simulink model "W05_S1"  (R2024b)
settings: Solver=ode4  StartTime=0  StopTime=T_final  FixedStep=h  RelTol=1e-3
values from neighbouring files (symbols this model uses):
  Delta = 8    [W05_S_expected.m]
  x0 = zeros(12,1);  x0(8) = V.y0;  assignin(b,'x0',x0)    [W05_S_expected.m]
undefined symbols (not defined in the file or in its folder): beta_c, k_neg, k_pos, Kd, Kp, law, mp, n_max, n_min, rp, V_c, WP_E, WP_N, X_ff, y_pont
settings Model: Creator=admin  LastModifiedBy=admin
settings DataIOCC: ReturnWorkspaceOutputs=off

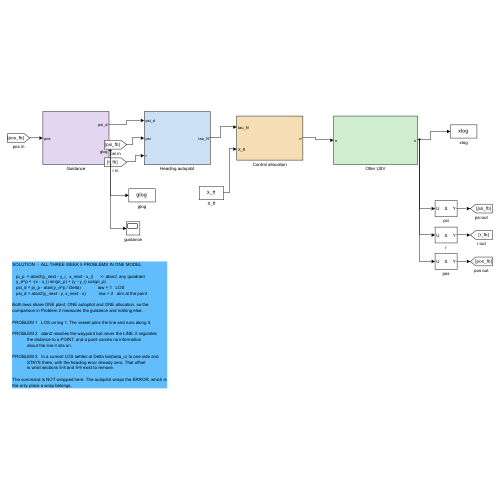
[thumbnail: Simulink's stored preview of the top-level diagram]
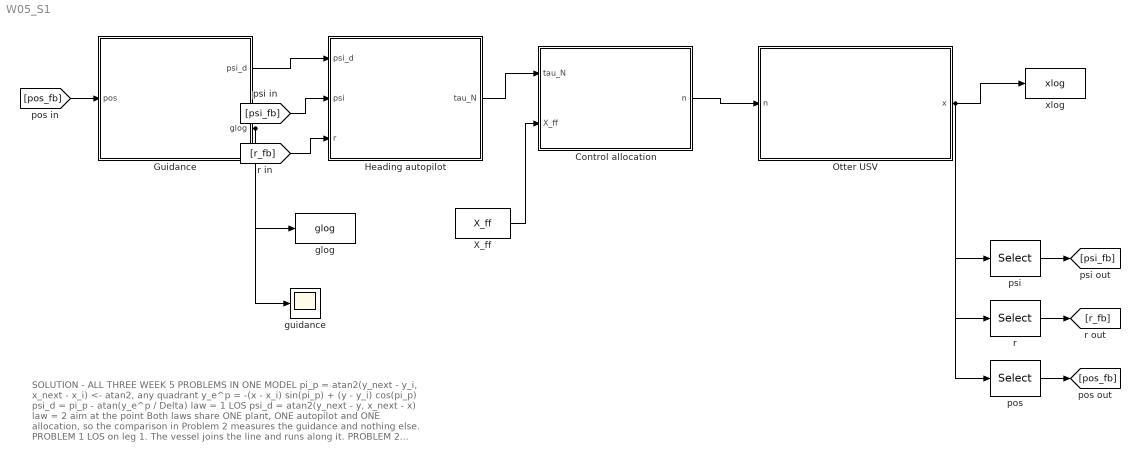
== system W05_S1 ==
  note: SOLUTION  -  ALL THREE WEEK 5 PROBLEMS IN ONE MODEL
      |
      |    pi_p  = atan2(y_next - y_i,  x_next - x_i)      <- atan2, any quadrant
      |    y_e^p = -(x - x_i) sin(pi_p) + (y - y_i) cos(pi_p)
      |    psi_d = pi_p - atan(y_e^p / Delta)              law = 1   LOS
      |    psi_d = atan2(y_next - y, x_next - x)           law = 2   aim at the point
      |
      | Both laws share ONE plant, ONE autopilot and ONE allocation, so the
      | comparison in Problem 2 measures the guidance and nothing else.
      |
      | PROBLEM 1   LOS on leg 1. The vessel joins the line and runs along it.
      |
      | PROBLEM 2   atan2 reaches the waypoint but never the LINE: it regulates
      |             the distance to a POINT, and a point carries no information
      |             about the line it sits on.
      |
      | PROBLEM 3   In a current LOS settles at Delta tan(beta_c) to one side and
      |             STAYS there, with the heading error already zero. That offset
      |             is what sections 5-8 and 5-9 exist to remove.
      |
      | The command is NOT wrapped here. The autopilot wraps the ERROR, which is
      | the only place a wrap belongs.
  Control allocation : Subsystem
  Guidance : Subsystem
  Heading autopilot : Subsystem
  Otter USV : Subsystem
  X_ff : Constant  Value=X_ff
  glog : ToWorkspace  VariableName=glog  SaveFormat=Structure With Time  SampleTime=-1
  guidance : Scope
  pos : Selector  InputPortWidth=12  IndexOptions=Index vector (dialog)  Indices=[7 8]  OutputSizes=1
  psi : Selector  InputPortWidth=12  IndexOptions=Index vector (dialog)  Indices=12  OutputSizes=1
  r : Selector  InputPortWidth=12  IndexOptions=Index vector (dialog)  Indices=6  OutputSizes=1
  xlog : ToWorkspace  VariableName=xlog  SaveFormat=Structure With Time  SampleTime=-1
  wires:
  Heading autopilot/1(tau_N) -> Control allocation/1(tau_N)
  X_ff/1 -> Control allocation/2(X_ff)
  Control allocation/1(n) -> Otter USV/1(n)
  Otter USV/1(x) -> xlog/1, psi/1, r/1, pos/1
  psi/1 -> [psi_fb]
  r/1 -> [r_fb]
  [psi_fb] -> Heading autopilot/2(psi)
  [r_fb] -> Heading autopilot/3(r)
  pos/1 -> [pos_fb]
  [pos_fb] -> Guidance/1(pos)
  Guidance/1(psi_d) -> Heading autopilot/1(psi_d)
  Guidance/2(glog) -> glog/1, guidance/1

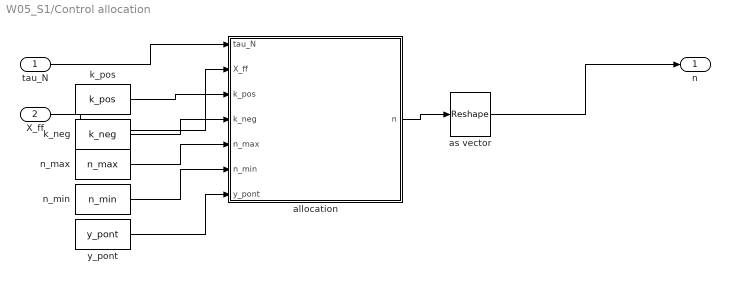
== system W05_S1/Control allocation ==
  tau_N : Inport
  X_ff : Inport  Port=2
  allocation : MATLAB Function  TreatAsAtomicUnit=on
  as vector : Reshape
  k_neg : Constant  Value=k_neg
  k_pos : Constant  Value=k_pos
  n_max : Constant  Value=n_max
  n_min : Constant  Value=n_min
  y_pont : Constant  Value=y_pont
  n : Outport
  wires:
  k_pos/1 -> allocation/3(k_pos)
  k_neg/1 -> allocation/4(k_neg)
  n_max/1 -> allocation/5(n_max)
  n_min/1 -> allocation/6(n_min)
  y_pont/1 -> allocation/7(y_pont)
  tau_N/1 -> allocation/1(tau_N)
  X_ff/1 -> allocation/2(X_ff)
  allocation/1(n) -> as vector/1
  as vector/1 -> n/1

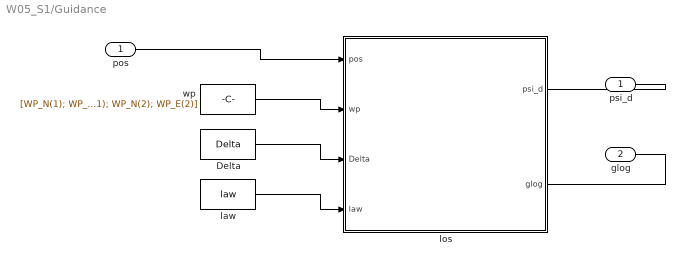
== system W05_S1/Guidance ==
  pos : Inport
  Delta : Constant  Value=Delta
  law : Constant  Value=law
  los : MATLAB Function  TreatAsAtomicUnit=on
  wp : Constant  Value=[WP_N(1); WP_E(1); WP_N(2); WP_E(2)]
  psi_d : Outport
  glog : Outport  Port=2
  wires:
  pos/1 -> los/1(pos)
  wp/1 -> los/2(wp)
  Delta/1 -> los/3(Delta)
  law/1 -> los/4(law)
  los/1(psi_d) -> psi_d/1
  los/2(glog) -> glog/1

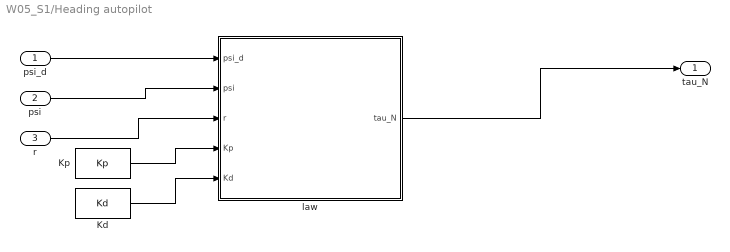
== system W05_S1/Heading autopilot ==
  psi_d : Inport
  psi : Inport  Port=2
  r : Inport  Port=3
  Kd : Constant  Value=Kd
  Kp : Constant  Value=Kp
  law : MATLAB Function  TreatAsAtomicUnit=on
  tau_N : Outport
  wires:
  Kp/1 -> law/4(Kp)
  Kd/1 -> law/5(Kd)
  psi_d/1 -> law/1(psi_d)
  psi/1 -> law/2(psi)
  r/1 -> law/3(r)
  law/1(tau_N) -> tau_N/1

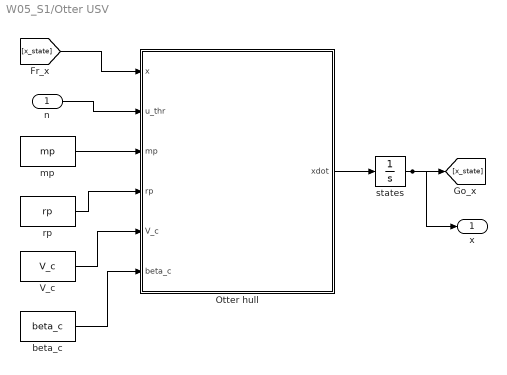
== system W05_S1/Otter USV ==
  n : Inport
  Otter hull : MATLAB Function  TreatAsAtomicUnit=on
  V_c : Constant  Value=V_c
  beta_c : Constant  Value=beta_c
  mp : Constant  Value=mp
  rp : Constant  Value=rp
  states : Integrator  InitialCondition=x0
  x : Outport
  wires:
  beta_c/1 -> Otter hull/6(beta_c)
  [x_state] -> Otter hull/1(x)
  n/1 -> Otter hull/2(u_thr)
  mp/1 -> Otter hull/3(mp)
  rp/1 -> Otter hull/4(rp)
  Otter hull/1(xdot) -> states/1
  V_c/1 -> Otter hull/5(V_c)
  states/1 -> [x_state], x/1

== matlab function W05_S1/Heading autopilot/law ==
  data: psi_d input; tau_N output double size=[1 1]; psi input; r input; Kp input; Kd input
function tau_N = law(psi_d, psi, r, Kp, Kd)
%#codegen
%LAW  Week 4's heading autopilot, unchanged.
%
%  tau_N = Kp ssa(psi_d - psi) - Kd r
%
%  The wrap is not optional here: guidance produces commands anywhere in
%  (-pi, pi], so the +-180 deg seam is crossed on almost every mission.
e = mod(psi_d - psi + pi, 2*pi) - pi;
tau_N = Kp*e - Kd*r;

== matlab function W05_S1/Guidance/los ==
  data: pos input; psi_d output; wp input; Delta input; law input; glog output
function [psi_d, glog] = los(pos, wp, Delta, law)
%#codegen
%LOS  Line-of-sight guidance on one straight leg.
%
%  pos   [x ; y] in {n} [m]
%  wp    [x_i ; y_i ; x_next ; y_next] — the active leg, in {n} [m]
%  law   1 = LOS, 2 = aim at the waypoint (atan2)
%
%  Returns psi_d [rad] and glog = [pi_p ; y_e_p ; psi_d].
x  = pos(1);      y  = pos(2);
xi = wp(1);       yi = wp(2);
xn = wp(3);       yn = wp(4);

%  The path-tangential angle MUST be atan2: a leg can point into any
%  quadrant, and the one-argument form folds two of them onto the others.
pi_p = atan2(yn - yi, xn - xi);

%  One rotation into the path frame gives BOTH errors. Only y_e is used
%  here; x_e is what the switching test of section F reads.
dx =  x - xi;   dy =  y - yi;
x_e =  dx*cos(pi_p) + dy*sin(pi_p);
y_e = -dx*sin(pi_p) + dy*cos(pi_p);

if law < 1.5
    %  Delta > 0 always, so the aim-point vector stays in the right
    %  half-plane of {p} and the one-argument atan is exact here.
    psi_d = pi_p - atan(y_e / Delta);
else
    psi_d = atan2(yn - y, xn - x);
end
glog = [pi_p; y_e; psi_d];

== matlab function W05_S1/Control allocation/allocation ==
  data: tau_N input; n output double size=[2 1]; X_ff input; k_pos input; k_neg input; n_max input; n_min input; y_pont input
function n = allocation(tau_N, X_ff, k_pos, k_neg, n_max, n_min, y_pont)
%#codegen
% Demanded surge force and yaw moment to two shaft speeds. Appendix A1.
T = [X_ff/2 + tau_N/(2*y_pont);
     X_ff/2 - tau_N/(2*y_pont)];
n = zeros(2,1);
for i = 1:2
    if T(i) >= 0
        ni =  sqrt( T(i) / k_pos);
    else
        ni = -sqrt(-T(i) / k_neg);
    end
    n(i) = min(max(ni, n_min), n_max);
end
end

== matlab function W05_S1/Otter USV/Otter hull ==
  data: x input; xdot output double size=[12 1]; u_thr input; mp input; rp input; V_c input; beta_c input
function xdot = otter_hull(x, u_thr, mp, rp, V_c, beta_c)
% Fossen's otter.m, called unchanged from Tools/MSS/VESSELS.
%
%   x       12 states, fed back from the integrator
%   u_thr   propeller shaft speeds [rad/s]
%
% otter.m is not written for code generation, so the call is extrinsic and
% xdot has to be pre-sized for Simulink to know the output width.
coder.extrinsic('otter');

xdot = zeros(12,1);
xdot = otter(x, u_thr, mp, rp, V_c, beta_c);
end
